simulink model "simulation_2"  (R2023b)
settings: Solver=VariableStepAuto  StartTime=0.0  StopTime=10.0  RelTol=1e-3
model workspace (MAT data in the model file):
  L = Simulink.Parameter
  L.Value = 50
  L.DataType = 'auto'
  L.DocUnits = 'm'
  L.Complexity = 'real'
  L.Dimensions = [1 1]
  a = Simulink.Parameter
  a.Value = 10
  a.DataType = 'auto'
  a.DocUnits = 'm'
  a.Complexity = 'real'
  a.Dimensions = [1 1]
  c = Simulink.Parameter
  c.Value = 340
  c.DataType = 'auto'
  c.DocUnits = 'm/s'
  c.Complexity = 'real'
  c.Dimensions = [1 1]
  n = Simulink.Parameter
  n.Value = Simulink.data.Expression
  n.Value.ExpressionString = "[2*pi*f*(L/c)]"
  n.DataType = 'auto'
  n.Complexity = 'real'
  n.Dimensions = -1
  v = 92.3997839291
settings Model: Creator=nurbi  LastModifiedBy=nurbi

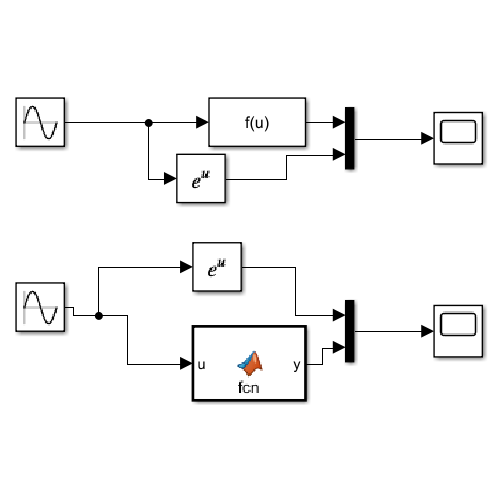
[thumbnail: Simulink's stored preview of the top-level diagram]
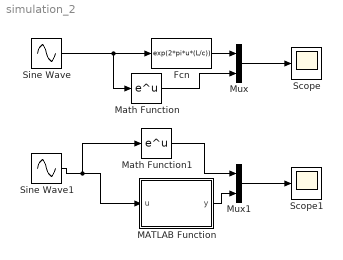
== system simulation_2 ==
  Fcn : Fcn  Expr=exp(2*pi*u*(L/c))
  MATLAB Function : MATLAB Function  TreatAsAtomicUnit=on
  Math Function : Math
  Math Function1 : Math
  Mux : Mux  Inputs=2
  Mux1 : Mux  Inputs=2
  Scope : Scope
  Scope1 : Scope
  Sine Wave : Sin  SampleTime=0
  Sine Wave1 : Sin  SampleTime=0
  wires:
  Mux/1 -> Scope/1
  Sine Wave/1 -> Fcn/1, Math Function/1
  Math Function/1 -> Mux/2
  Sine Wave1/1 -> Math Function1/1, MATLAB Function/1(u)
  Mux1/1 -> Scope1/1
  MATLAB Function/1(y) -> Mux1/2
  Math Function1/1 -> Mux1/1
  Fcn/1 -> Mux/1

== matlab function simulation_2/MATLAB Function ==
  data: u input; y output
function y = fcn(u)

L = 50;
c = 340;
f = u;

y = exp(2*pi*f*(L/c));
